simulink model "exampleMinStopTime"  (Simulink 7.6)
settings: Solver=ode45  StartTime=0.0  StopTime=30  RelTol=1e-3
settings Model: Creator=drhf  LastModifiedBy=awohlfei
settings CodeAppCC: CustomSymbolStrType=$N$R$M_T

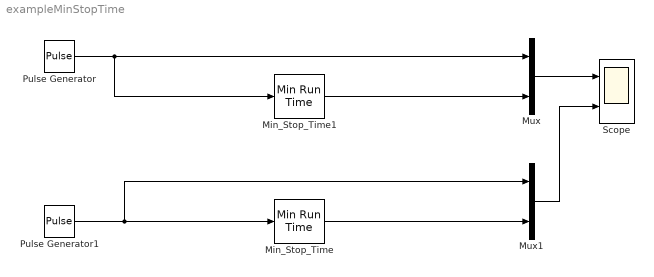
== system exampleMinStopTime ==
  Min_Stop_Time : Reference  SystemSampleTime=-1  tminstop=15
  Min_Stop_Time1 : Reference  SystemSampleTime=-1  tminstop=15
  Mux : Mux  Inputs=2
  Mux1 : Mux  Inputs=2
  Pulse Generator : DiscretePulseGenerator  PulseType=Time based  Amplitude=2  Period=10  PulseWidth=80
  Pulse Generator1 : DiscretePulseGenerator  PulseType=Time based  Amplitude=2  Period=8  PulseWidth=5
  Scope : Scope  NumInputPorts=2
      settings: YMin=-5~-5  YMax=5~5
  wires:
  Pulse Generator/1 -> Mux/1, Min_Stop_Time1/1
  Mux/1 -> Scope/1
  Min_Stop_Time1/1 -> Mux/2
  Pulse Generator1/1 -> Mux1/1, Min_Stop_Time/1
  Min_Stop_Time/1 -> Mux1/2
  Mux1/1 -> Scope/2
